simulink model "SimulationWithMotorAndGearbox"  (R2023a)
settings: configuration reference "SharedConfig" (kept outside this file)
undefined symbols (not defined in the file): Analyse, config_gearbox, config_motor, GB, gearbox_map, k_FW, motormap, motormap2
libraries: simulink x2
settings Model: PauseTimes=35  Creator=maximilian.tschochne  LastModifiedBy=ge49hus
settings ConfigSetRef: SourceName=SharedConfig  SourceLocation=Base Workspace

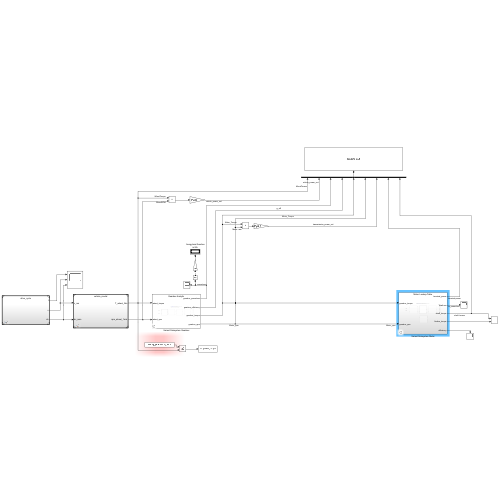
[thumbnail: Simulink's stored preview of the top-level diagram]
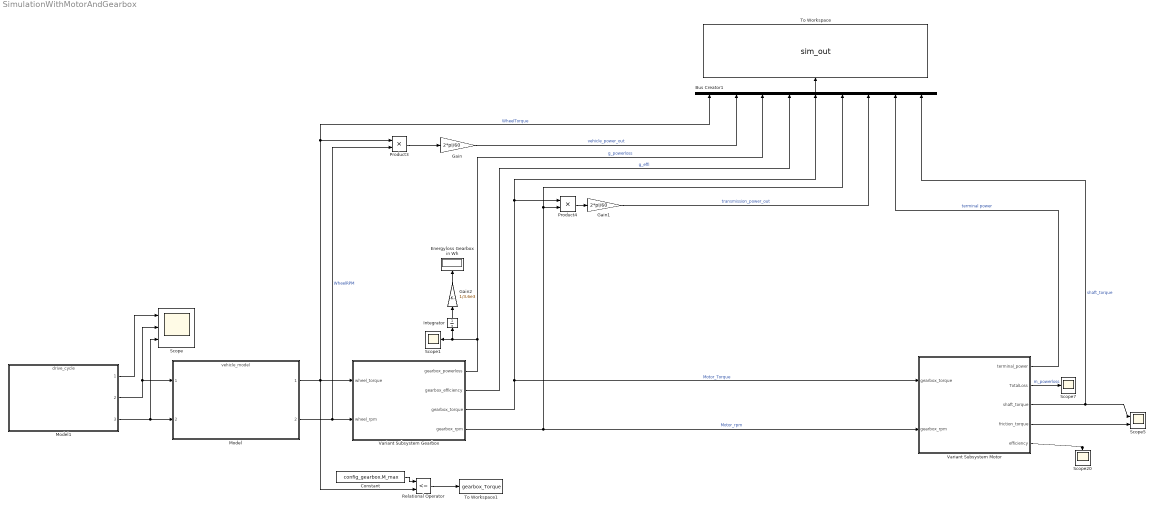
== system SimulationWithMotorAndGearbox ==
  Bus Creator1 : BusCreator  Inputs=9
  Constant : Constant  Value=config_gearbox.M_max
  Energyloss Gearbox in Wh : Display
  Gain : Gain  Gain=2*pi/60
  Gain1 : Gain  Gain=2*pi/60
  Gain2 : Gain  Gain=1/3.6e3
  Integrator : Integrator
  Model : ModelReference  ModelNameDialog=vehicle_model.slx  SimulationMode=Normal  ModelReferenceVersion=2.0
  Model1 : ModelReference  ModelNameDialog=drive_cycle.slx  SimulationMode=Normal  ModelReferenceVersion=1.0
  Product3 : Product
  Product4 : Product
  Relational Operator : RelationalOperator  Operator=<=  OutDataTypeStr=boolean  RndMeth=Simplest  InputSameDT=off
  Scope : Scope  NumInputPorts=3
  Scope1 : Scope
  Scope20 : Scope
  Scope5 : Scope  NumInputPorts=2
  Scope7 : Scope
  To Workspace : ToWorkspace  VariableName=sim_out  SaveFormat=Timeseries  SampleTime=-1
  To Workspace1 : ToWorkspace  VariableName=gearbox_Torque  SaveFormat=Timeseries  SampleTime=-1
  Variant Subsystem Gearbox : Subsystem  Variant=on
  Variant Subsystem Motor : Subsystem  Variant=on
  wires:
  Model1/1 -> Scope/1
  Model1/2 -> Scope/2, Model/1
  Model1/3 -> Scope/3, Model/2
  Bus Creator1/1 -> To Workspace/1
  Gain/1 -> Bus Creator1/2  "vehicle_power_out"
  Gain1/1 -> Bus Creator1/7  "transmission_power_out"
  Model/2 -> Product3/2, Variant Subsystem Gearbox/2(wheel_rpm)  "WheelRPM"
  Model/1 -> Variant Subsystem Gearbox/1(wheel_torque), Relational Operator/2, Bus Creator1/1, Product3/1  "WheelTorque"
  Product3/1 -> Gain/1
  Product4/1 -> Gain1/1
  Variant Subsystem Gearbox/1(gearbox_powerloss) -> Bus Creator1/3, Integrator/1, Scope1/1  "g_powerloss"
  Variant Subsystem Gearbox/2(gearbox_efficiency) -> Bus Creator1/4  "g_effi"
  Integrator/1 -> Gain2/1
  Gain2/1 -> Energyloss Gearbox in Wh/1
  Relational Operator/1 -> To Workspace1/1
  Constant/1 -> Relational Operator/1
  Variant Subsystem Gearbox/3(gearbox_torque) -> Bus Creator1/5, Product4/1, Variant Subsystem Motor/1(gearbox_torque)  "Motor_Torque"
  Variant Subsystem Gearbox/4(gearbox_rpm) -> Variant Subsystem Motor/2(gearbox_rpm), Bus Creator1/6, Product4/2  "Motor_rpm"
  Variant Subsystem Motor/3(shaft_torque) -> Bus Creator1/9, Scope5/1  "shaft_torque"
  Variant Subsystem Motor/5(efficiency) -> Scope20/1
  Variant Subsystem Motor/1(terminal_power) -> Bus Creator1/8  "terminal power"
  Variant Subsystem Motor/4(friction_torque) -> Scope5/2
  Variant Subsystem Motor/2(TotalLoss) -> Scope7/1  "m_powerloss"

== system SimulationWithMotorAndGearbox/Variant Subsystem Gearbox ==
  note: 1) Add Subsystem or Model blocks as valid variant choices.
      | 2) You cannot connect blocks at this level. At simulation, connectivity is automatically
      | determined, based on the active variant and port name matching.
  wheel_torque : Inport
  wheel_rpm : Inport  Port=2
  Gearbox Analytic : Subsystem  VariantControl="GB_Mode == \"Analytic\""
  Gearbox Const : Subsystem  VariantControl="GB_Mode == \"Const\""
  Gearbox Lookup-Table : Subsystem  VariantControl="GB_Mode == \"Lookup\""
  Gearbox Simple : Subsystem  VariantControl="GB_Mode == \"Simple\""
  gearbox_powerloss : Outport
  gearbox_efficiency : Outport  Port=2
  gearbox_torque : Outport  Port=3
  gearbox_rpm : Outport  Port=4

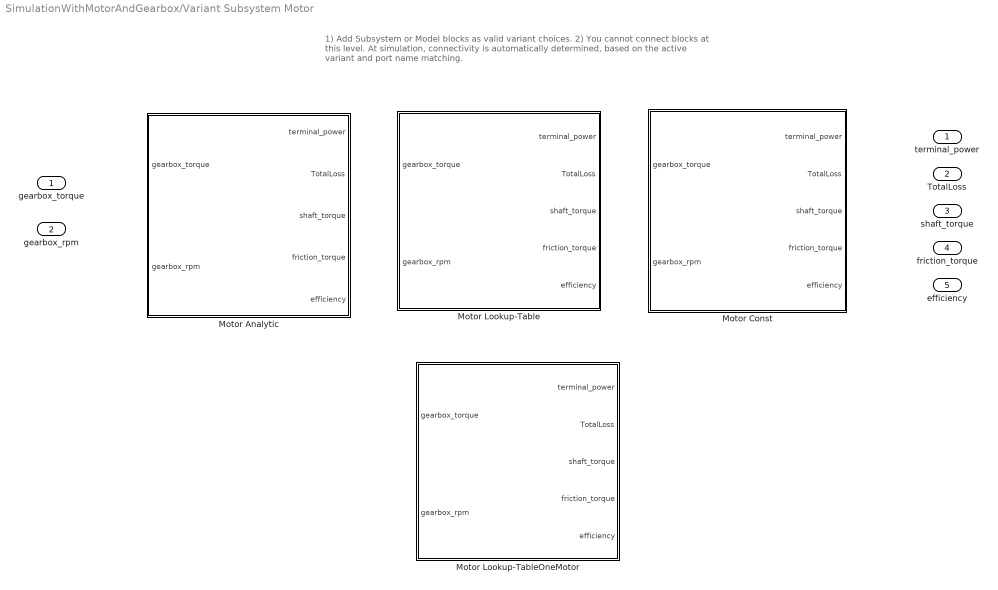
== system SimulationWithMotorAndGearbox/Variant Subsystem Motor ==
  note: 1) Add Subsystem or Model blocks as valid variant choices.
      | 2) You cannot connect blocks at this level. At simulation, connectivity is automatically
      | determined, based on the active variant and port name matching.
  gearbox_torque : Inport
  gearbox_rpm : Inport  Port=2
  Motor Analytic : Subsystem  VariantControl="Motor_Mode == \"Analytic\""
  Motor Const : Subsystem  VariantControl="Motor_Mode == \"Const\""
  Motor Lookup-Table : Subsystem  VariantControl="Motor_Mode == \"Lookup\""
  Motor Lookup-TableOneMotor : Subsystem  VariantControl="Motor_Mode == \"LookupOneMotor\""
  terminal_power : Outport
  TotalLoss : Outport  Port=2
  shaft_torque : Outport  Port=3
  friction_torque : Outport  Port=4
  efficiency : Outport  Port=5

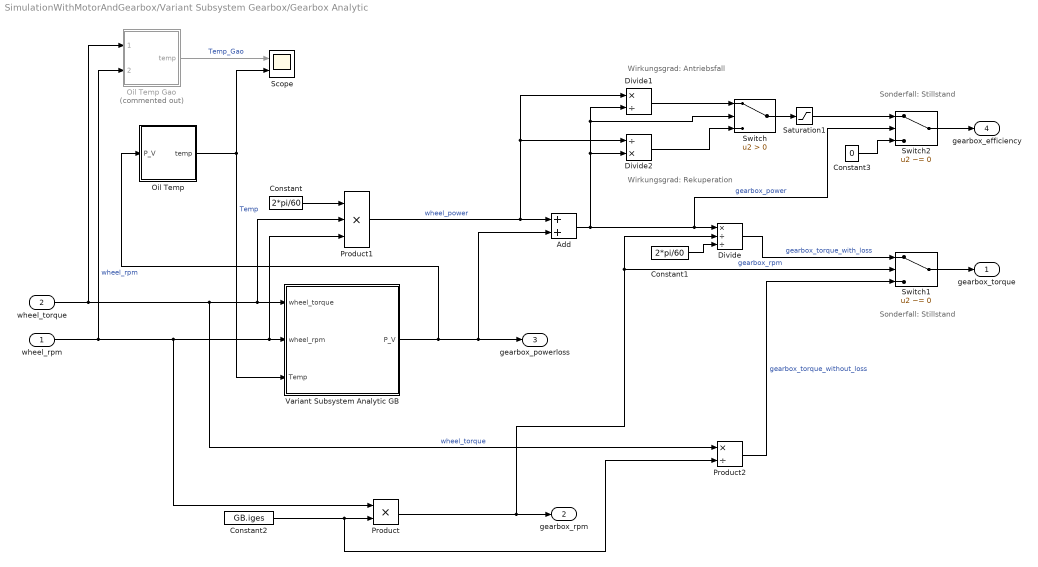
== system SimulationWithMotorAndGearbox/Variant Subsystem Gearbox/Gearbox Analytic ==
  note: Wirkungsgrad:
      | Antriebsfall
  note: Sonderfall: Stillstand
  note: Sonderfall: Stillstand
  note: Wirkungsgrad:
      | Rekuperation
  wheel_rpm : Inport
  wheel_torque : Inport  Port=2
  Add : Sum
  Constant : Constant  Value=2*pi/60
  Constant1 : Constant  Value=2*pi/60
  Constant2 : Constant  Value=GB.iges
  Constant3 : Constant  Value=0
  Divide : Product  Inputs=*//
  Divide1 : Product  Inputs=*/
  Divide2 : Product  Inputs=/*
  Oil Temp : Subsystem
  Oil Temp Gao : Subsystem  Commented=on
  Product : Product
  Product1 : Product  Inputs=3
  Product2 : Product  Inputs=*/
  Saturation1 : Saturate  UpperLimit=inf  LowerLimit=0
  Scope : Scope  NumInputPorts=2
  Switch : Switch  Criteria=u2 > Threshold  SaturateOnIntegerOverflow=off  InputSameDT=off
  Switch1 : Switch  Criteria=u2 ~= 0  SaturateOnIntegerOverflow=off  InputSameDT=off
  Switch2 : Switch  Criteria=u2 ~= 0  SaturateOnIntegerOverflow=off  InputSameDT=off
  Variant Subsystem Analytic GB : Subsystem  Variant=on
  gearbox_torque : Outport
  gearbox_rpm : Outport  Port=2
  gearbox_powerloss : Outport  Port=3
  gearbox_efficiency : Outport  Port=4
  wires:
  wheel_torque/1 -> Variant Subsystem Analytic GB/1(wheel_torque), Product1/2, Product2/1, Oil Temp Gao/1(T_wheel)  "wheel_torque"
  wheel_rpm/1 -> Product/1, Variant Subsystem Analytic GB/2(wheel_rpm), Product1/3, Oil Temp Gao/2(rpm_wheel)  "wheel_rpm"
  Variant Subsystem Analytic GB/1(P_V) -> Oil Temp/1(P_V), Add/2, gearbox_powerloss/1
  Constant2/1 -> Product2/2, Product/2
  Product/1 -> Switch1/2, Divide/2, gearbox_rpm/1  "gearbox_rpm"
  Constant/1 -> Product1/1
  Product1/1 -> Divide2/1, Divide1/1, Add/1  "wheel_power"
  Add/1 -> Divide2/2, Switch/2, Divide1/2, Switch2/2, Divide/1  "gearbox_power"
  Constant1/1 -> Divide/3
  Divide/1 -> Switch1/1  "gearbox_torque_with_loss"
  Switch/1 -> Saturation1/1
  Divide2/1 -> Switch/3
  Switch1/1 -> gearbox_torque/1
  Product2/1 -> Switch1/3  "gearbox_torque_without_loss"
  Switch2/1 -> gearbox_efficiency/1
  Constant3/1 -> Switch2/3
  Divide1/1 -> Switch/1
  Oil Temp Gao/1(temp) -> Scope/1  "Temp_Gao"
  Oil Temp/1(temp) -> Scope/2, Variant Subsystem Analytic GB/3(Temp)  "Temp"
  Saturation1/1 -> Switch2/1

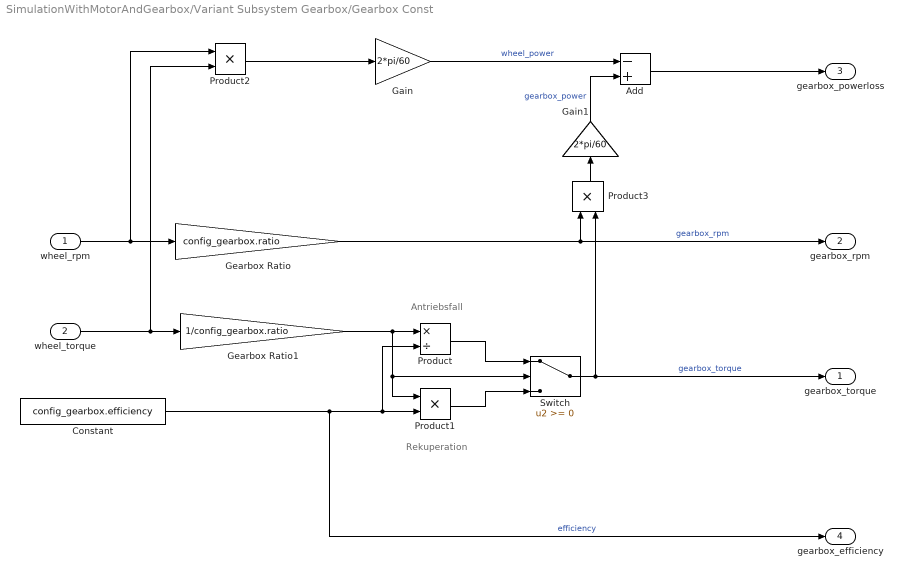
== system SimulationWithMotorAndGearbox/Variant Subsystem Gearbox/Gearbox Const ==
  note: Rekuperation
  note: Antriebsfall
  wheel_rpm : Inport
  wheel_torque : Inport  Port=2
  Add : Sum  Inputs=-+
  Constant : Constant  Value=config_gearbox.efficiency
  Gain : Gain  Gain=2*pi/60
  Gain1 : Gain  Gain=2*pi/60
  Gearbox Ratio : Gain  Gain=config_gearbox.ratio
  Gearbox Ratio1 : Gain  Gain=1/config_gearbox.ratio
  Product : Product  Inputs=*/
  Product1 : Product  Inputs=**
  Product2 : Product
  Product3 : Product
  Switch : Switch  SaturateOnIntegerOverflow=off  InputSameDT=off
  gearbox_torque : Outport
  gearbox_rpm : Outport  Port=2
  gearbox_powerloss : Outport  Port=3
  gearbox_efficiency : Outport  Port=4
  wires:
  wheel_rpm/1 -> Product2/1, Gearbox Ratio/1
  Gearbox Ratio/1 -> gearbox_rpm/1, Product3/1  "gearbox_rpm"
  wheel_torque/1 -> Product2/2, Gearbox Ratio1/1
  Gearbox Ratio1/1 -> Product1/1, Switch/2, Product/1
  Constant/1 -> gearbox_efficiency/1, Product1/2, Product/2  "efficiency"
  Product/1 -> Switch/1
  Product1/1 -> Switch/3
  Switch/1 -> gearbox_torque/1, Product3/2  "gearbox_torque"
  Product2/1 -> Gain/1
  Add/1 -> gearbox_powerloss/1
  Product3/1 -> Gain1/1
  Gain/1 -> Add/1  "wheel_power"
  Gain1/1 -> Add/2  "gearbox_power"

== system SimulationWithMotorAndGearbox/Variant Subsystem Gearbox/Gearbox Lookup-Table ==
  wheel_rpm : Inport
  wheel_torque : Inport  Port=2
  Oil Temp : Subsystem
  Oil Temp Gao : Subsystem  Commented=on
  Scope : Scope  Commented=on  NumInputPorts=2
  Variant Subsystem : Subsystem  Variant=on
  gearbox_torque : Outport
  gearbox_rpm : Outport  Port=2
  gearbox_powerloss : Outport  Port=3
  gearbox_efficiency : Outport  Port=4
  wires:
  Oil Temp Gao/1(temp) -> Scope/2
  wheel_torque/1 -> Oil Temp Gao/1(T_wheel), Variant Subsystem/1(wheel_torque)  "wheel_torque"
  wheel_rpm/1 -> Oil Temp Gao/2(rpm_wheel), Variant Subsystem/2(wheel_rpm)  "wheel_rpm"
  Variant Subsystem/4(gearbox_torque) -> gearbox_torque/1
  Variant Subsystem/1(loss_lockup) -> Oil Temp/1(P_V), gearbox_powerloss/1
  Variant Subsystem/3(gearbox_rpm) -> gearbox_rpm/1
  Variant Subsystem/2(gearbox_efficiency) -> gearbox_efficiency/1
  Oil Temp/1(temp) -> Scope/1, Variant Subsystem/3(Temp)

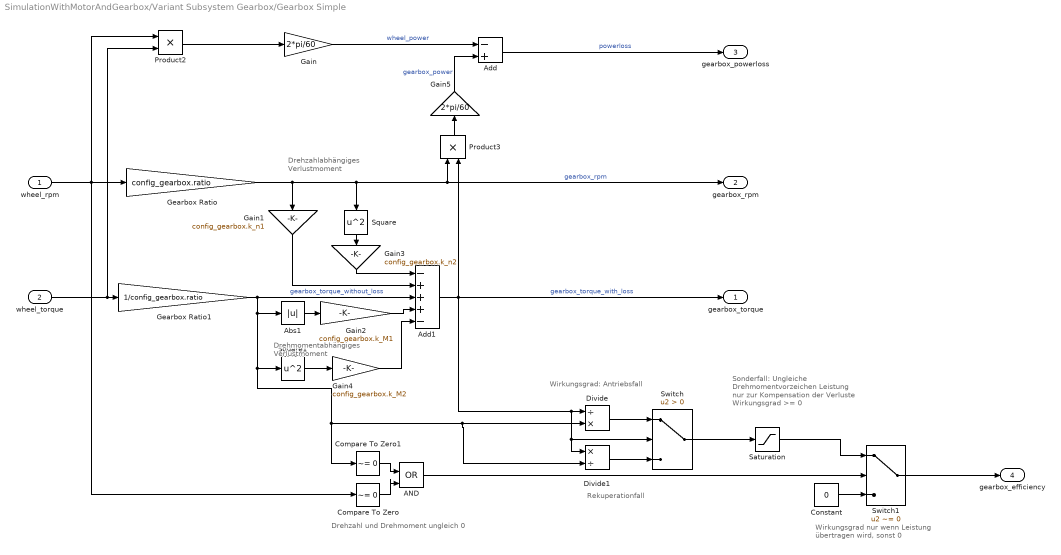
== system SimulationWithMotorAndGearbox/Variant Subsystem Gearbox/Gearbox Simple ==
  note: Rekuperationfall
  note: Sonderfall: Ungleiche Drehmomentvorzeichen
      | Leistung nur zur Kompensation der Verluste
      | Wirkungsgrad >= 0
  note: Drehzahl und Drehmoment ungleich 0
  note: Drehmomentabhängiges
      | Verlustmoment
  note: Drehzahlabhängiges
      | Verlustmoment
  note: Wirkungsgrad nur wenn Leistung
      | übertragen wird, sonst 0
  note: Wirkungsgrad: Antriebsfall
  wheel_rpm : Inport
  wheel_torque : Inport  Port=2
  AND : Logic  Operator=OR  IconShape=distinctive  AllPortsSameDT=off  OutDataTypeStr=boolean
  Abs1 : Abs  SaturateOnIntegerOverflow=off
  Add : Sum  Inputs=-+
  Add1 : Sum  Inputs=-+++-
  Compare To Zero : simulink/Logic and Bit Operations/Compare To Zero  relop=~=  OutDataTypeStr=boolean
  Compare To Zero1 : simulink/Logic and Bit Operations/Compare To Zero  relop=~=  OutDataTypeStr=boolean
  Constant : Constant  Value=0
  Divide : Product  Inputs=/*
  Divide1 : Product  Inputs=*/
  Gain : Gain  Gain=2*pi/60
  Gain1 : Gain  Gain=config_gearbox.k_n1
  Gain2 : Gain  Gain=config_gearbox.k_M1
  Gain3 : Gain  Gain=config_gearbox.k_n2
  Gain4 : Gain  Gain=config_gearbox.k_M2
  Gain5 : Gain  Gain=2*pi/60
  Gearbox Ratio : Gain  Gain=config_gearbox.ratio
  Gearbox Ratio1 : Gain  Gain=1/config_gearbox.ratio
  Product2 : Product
  Product3 : Product
  Saturation : Saturate  UpperLimit=inf  LowerLimit=0
  Square : Math  Operator=square
  Square1 : Math  Operator=square
  Switch : Switch  Criteria=u2 > Threshold  SaturateOnIntegerOverflow=off  InputSameDT=off
  Switch1 : Switch  Criteria=u2 ~= 0  SaturateOnIntegerOverflow=off  InputSameDT=off
  gearbox_torque : Outport
  gearbox_rpm : Outport  Port=2
  gearbox_powerloss : Outport  Port=3
  gearbox_efficiency : Outport  Port=4
  wires:
  Product3/1 -> Gain5/1
  Add/1 -> gearbox_powerloss/1  "powerloss"
  Add1/1 -> Product3/2, gearbox_torque/1, Switch/2, Divide1/1, Divide/1  "gearbox_torque_with_loss"
  wheel_torque/1 -> Product2/2, Gearbox Ratio1/1
  Gearbox Ratio/1 -> Square/1, Product3/1, gearbox_rpm/1, Gain1/1  "gearbox_rpm"
  wheel_rpm/1 -> Compare To Zero/1, Gearbox Ratio/1, Product2/1
  Gearbox Ratio1/1 -> Abs1/1, Square1/1, Compare To Zero1/1, Divide1/2, Divide/2, Add1/3  "gearbox_torque_without_loss"
  Gain1/1 -> Add1/2
  Gain2/1 -> Add1/4
  Abs1/1 -> Gain2/1
  Divide/1 -> Switch/1
  Switch/1 -> Saturation/1
  Divide1/1 -> Switch/3
  Constant/1 -> Switch1/3
  Gain3/1 -> Add1/1
  Square/1 -> Gain3/1
  Switch1/1 -> gearbox_efficiency/1
  Square1/1 -> Gain4/1
  Gain4/1 -> Add1/5
  Compare To Zero1/1 -> AND/1
  Compare To Zero/1 -> AND/2
  AND/1 -> Switch1/2
  Product2/1 -> Gain/1
  Gain/1 -> Add/1  "wheel_power"
  Gain5/1 -> Add/2  "gearbox_power"
  Saturation/1 -> Switch1/1

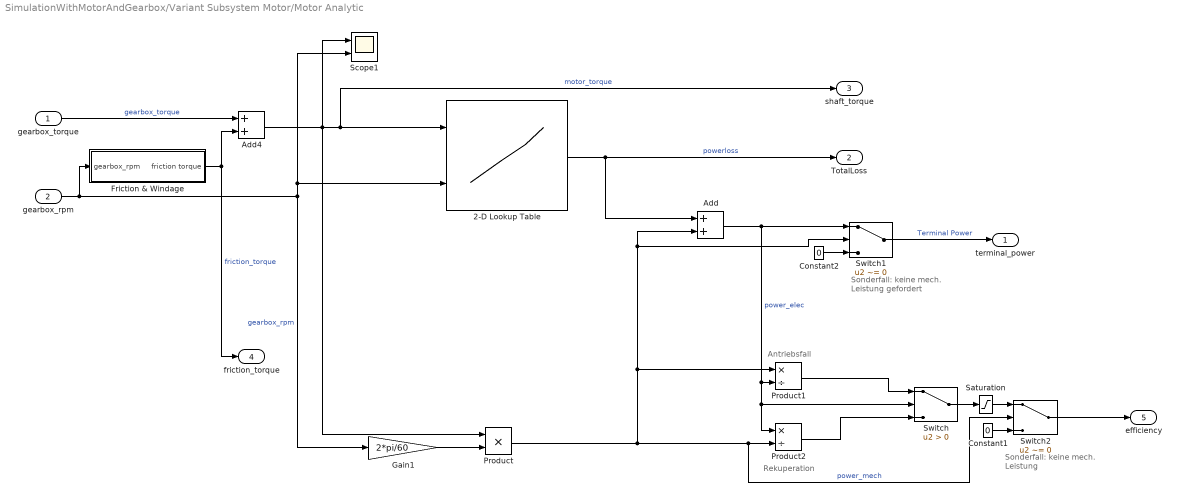
== system SimulationWithMotorAndGearbox/Variant Subsystem Motor/Motor Analytic ==
  note: Sonderfall:
      | keine mech. Leistung
  note: Antriebsfall
  note: Rekuperation
  note: Sonderfall: keine mech.
      | Leistung gefordert
  gearbox_torque : Inport
  gearbox_rpm : Inport  Port=2
  2-D Lookup Table : Lookup_n-D  BreakpointsForDimension1=Analyse.Betriebsdaten.M_vec(end:-1:1)  BreakpointsForDimension2=Analyse.Betriebsdaten.n_m_mesh(Analyse.Optionen.M_tics,:)  Table=Analyse.Verluste.P_vges_mesh(end:-1:1,:)  InternalRulePriority=Speed  RndMeth=Simplest
      settings: InputPortMap=u0,u1
  Add : Sum
  Add4 : Sum
  Constant1 : Constant  Value=0
  Constant2 : Constant  Value=0
  Friction & Windage : Subsystem
  Gain1 : Gain  Gain=2*pi/60
  Product : Product
  Product1 : Product  Inputs=*/
  Product2 : Product  Inputs=*/
  Saturation : Saturate  UpperLimit=inf  LowerLimit=0
  Scope1 : Scope  NumInputPorts=2
  Switch : Switch  Criteria=u2 > Threshold  SaturateOnIntegerOverflow=off  InputSameDT=off
  Switch1 : Switch  Criteria=u2 ~= 0  SaturateOnIntegerOverflow=off  InputSameDT=off
  Switch2 : Switch  Criteria=u2 ~= 0  SaturateOnIntegerOverflow=off  InputSameDT=off
  terminal_power : Outport
  TotalLoss : Outport  Port=2
  shaft_torque : Outport  Port=3
  friction_torque : Outport  Port=4
  efficiency : Outport  Port=5
  wires:
  gearbox_rpm/1 -> Friction & Windage/1(gearbox_rpm), Scope1/2, 2-D Lookup Table/2, Gain1/1  "gearbox_rpm"
  2-D Lookup Table/1 -> Add/1, TotalLoss/1  "powerloss"
  Product/1 -> Switch2/2, Product2/2, Switch1/2, Add/2, Product1/1  "power_mech"
  Add/1 -> Switch1/1, Product2/1, Switch/2, Product1/2  "power_elec"
  Product2/1 -> Switch/3
  Add4/1 -> Scope1/1, Product/1, shaft_torque/1, 2-D Lookup Table/1  "motor_torque"
  Switch2/1 -> efficiency/1
  Gain1/1 -> Product/2
  Constant2/1 -> Switch1/3
  Switch1/1 -> terminal_power/1  "Terminal Power"
  Product1/1 -> Switch/1
  gearbox_torque/1 -> Add4/1  "gearbox_torque"
  Friction & Windage/1(friction torque) -> friction_torque/1, Add4/2  "friction_torque"
  Switch/1 -> Saturation/1
  Constant1/1 -> Switch2/3
  Saturation/1 -> Switch2/1

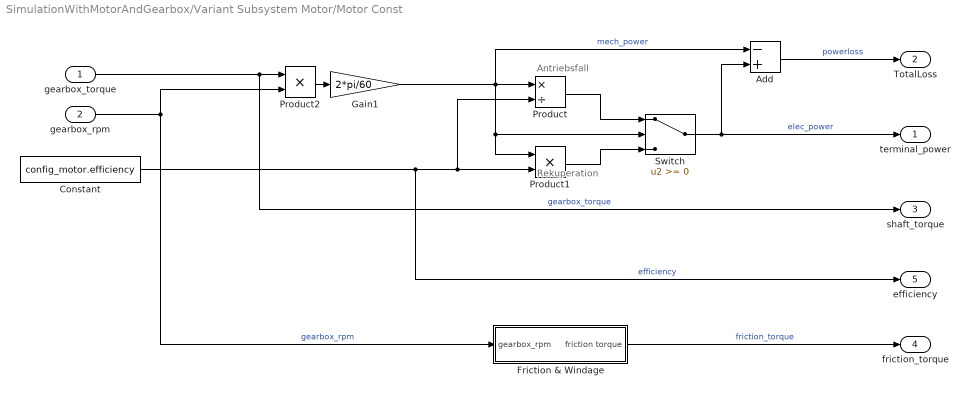
== system SimulationWithMotorAndGearbox/Variant Subsystem Motor/Motor Const ==
  note: Rekuperation
  note: Antriebsfall
  gearbox_torque : Inport
  gearbox_rpm : Inport  Port=2
  Add : Sum  Inputs=-+
  Constant : Constant  Value=config_motor.efficiency
  Friction & Windage : Subsystem
  Gain1 : Gain  Gain=2*pi/60
  Product : Product  Inputs=*/
  Product1 : Product  Inputs=**
  Product2 : Product
  Switch : Switch  SaturateOnIntegerOverflow=off  InputSameDT=off
  terminal_power : Outport
  TotalLoss : Outport  Port=2
  shaft_torque : Outport  Port=3
  friction_torque : Outport  Port=4
  efficiency : Outport  Port=5
  wires:
  Product2/1 -> Gain1/1
  Constant/1 -> efficiency/1, Product1/2, Product/2  "efficiency"
  Product/1 -> Switch/1
  Product1/1 -> Switch/3
  Add/1 -> TotalLoss/1  "powerloss"
  Switch/1 -> terminal_power/1, Add/2  "elec_power"
  gearbox_rpm/1 -> Friction & Windage/1(gearbox_rpm), Product2/2  "gearbox_rpm"
  Gain1/1 -> Add/1, Product1/1, Switch/2, Product/1  "mech_power"
  gearbox_torque/1 -> Product2/1, shaft_torque/1  "gearbox_torque"
  Friction & Windage/1(friction torque) -> friction_torque/1  "friction_torque"

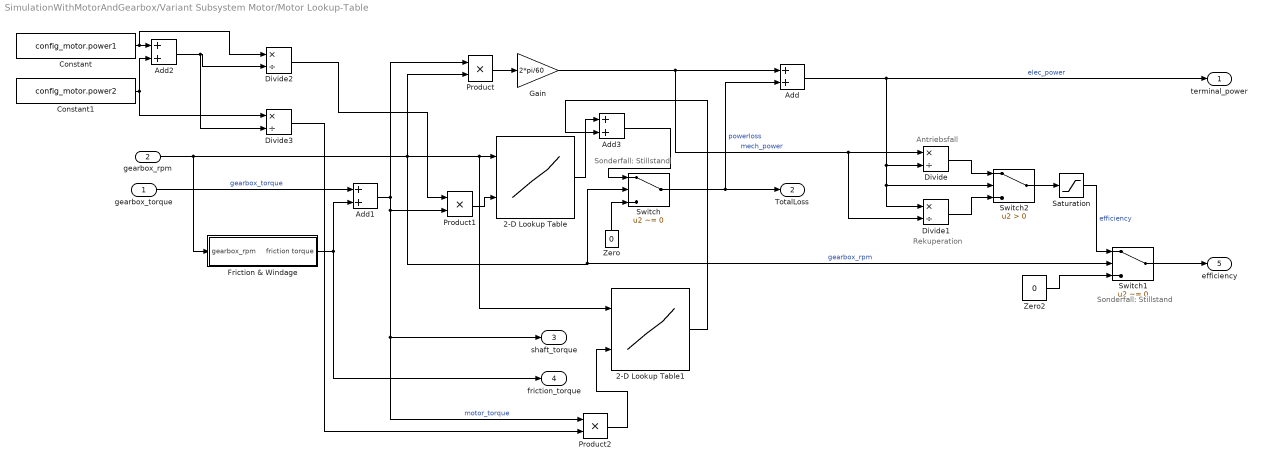
== system SimulationWithMotorAndGearbox/Variant Subsystem Motor/Motor Lookup-Table ==
  note: Sonderfall: Stillstand
  note: Rekuperation
  note: Antriebsfall
  note: Sonderfall: Stillstand
  gearbox_torque : Inport
  gearbox_rpm : Inport  Port=2
  2-D Lookup Table : Lookup_n-D  BreakpointsForDimension1=motormap.nVec  BreakpointsForDimension2=motormap.MVec  Table=motormap.Loss  InternalRulePriority=Speed  RndMeth=Simplest
      settings: InputPortMap=u0,u1
  2-D Lookup Table1 : Lookup_n-D  BreakpointsForDimension1=motormap2.nVec  BreakpointsForDimension2=motormap2.MVec  Table=motormap2.Loss  InternalRulePriority=Speed  RndMeth=Simplest
      settings: InputPortMap=u0,u1
  Add{,1..3} (4 alike) : Sum
  Constant : Constant  Value=config_motor.power1
  Constant1 : Constant  Value=config_motor.power2
  Divide{,1..3} (4 alike) : Product  Inputs=*/
  Friction & Windage : Subsystem
  Gain : Gain  Gain=2*pi/60
  Product : Product
  Product1 : Product
  Product2 : Product
  Saturation : Saturate  UpperLimit=inf  LowerLimit=0
  Switch : Switch  Criteria=u2 ~= 0  Threshold=1  SaturateOnIntegerOverflow=off  InputSameDT=off
  Switch1 : Switch  Criteria=u2 ~= 0  SaturateOnIntegerOverflow=off  InputSameDT=off
  Switch2 : Switch  Criteria=u2 > Threshold  SaturateOnIntegerOverflow=off  InputSameDT=off
  Zero : Constant  Value=0  OutDataTypeStr=Inherit: Inherit via back propagation
  Zero2 : Constant  Value=0  OutDataTypeStr=Inherit: Inherit via back propagation
  terminal_power : Outport
  TotalLoss : Outport  Port=2
  shaft_torque : Outport  Port=3
  friction_torque : Outport  Port=4
  efficiency : Outport  Port=5
  wires:
  gearbox_torque/1 -> Add1/1  "gearbox_torque"
  2-D Lookup Table/1 -> Add3/1
  Product/1 -> Gain/1
  Gain/1 -> Divide/1, Divide1/2, Add/1  "mech_power"
  Switch/1 -> TotalLoss/1, Add/2  "powerloss"
  Zero/1 -> Switch/3
  Add/1 -> Switch2/2, Divide1/1, Divide/2, terminal_power/1  "elec_power"
  Switch1/1 -> efficiency/1
  Zero2/1 -> Switch1/3
  Switch2/1 -> Saturation/1
  Divide/1 -> Switch2/1
  Divide1/1 -> Switch2/3
  Saturation/1 -> Switch1/1  "efficiency"
  gearbox_rpm/1 -> 2-D Lookup Table1/1, 2-D Lookup Table/1, Switch1/2, Switch/2, Product/2, Friction & Windage/1(gearbox_rpm)  "gearbox_rpm"
  Add1/1 -> Product1/2, Product2/1, shaft_torque/1, Product/1  "motor_torque"
  Friction & Windage/1(friction torque) -> Add1/2, friction_torque/1
  Constant/1 -> Divide2/1, Add2/1
  Constant1/1 -> Add2/2, Divide3/1
  Add2/1 -> Divide3/2, Divide2/2
  Divide2/1 -> Product1/1
  Product1/1 -> 2-D Lookup Table/2
  Product2/1 -> 2-D Lookup Table1/2
  Divide3/1 -> Product2/2
  2-D Lookup Table1/1 -> Add3/2
  Add3/1 -> Switch/1

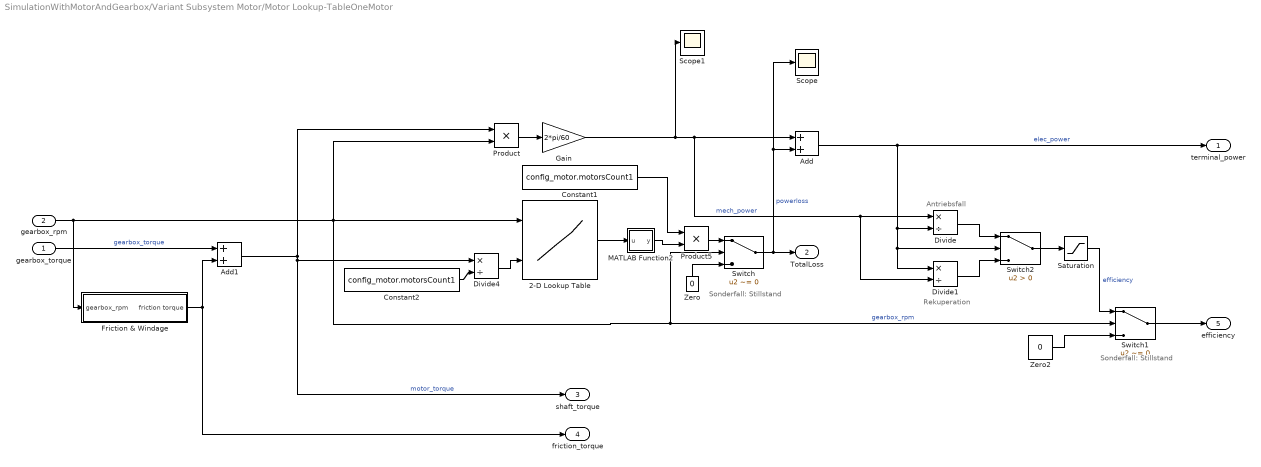
== system SimulationWithMotorAndGearbox/Variant Subsystem Motor/Motor Lookup-TableOneMotor ==
  note: Sonderfall: Stillstand
  note: Rekuperation
  note: Antriebsfall
  note: Sonderfall: Stillstand
  gearbox_torque : Inport
  gearbox_rpm : Inport  Port=2
  2-D Lookup Table : Lookup_n-D  BreakpointsForDimension1=motormap.nVec  BreakpointsForDimension2=motormap.MVec  Table=motormap.Loss  InternalRulePriority=Speed  RndMeth=Simplest
      settings: InputPortMap=u0,u1
  Add : Sum
  Add1 : Sum
  Constant1 : Constant  Value=config_motor.motorsCount1
  Constant2 : Constant  Value=config_motor.motorsCount1
  Divide : Product  Inputs=*/
  Divide1 : Product  Inputs=*/
  Divide4 : Product  Inputs=*/
  Friction & Windage : Subsystem
  Gain : Gain  Gain=2*pi/60
  MATLAB Function2 : MATLAB Function  TreatAsAtomicUnit=on
  Product : Product
  Product5 : Product
  Saturation : Saturate  UpperLimit=inf  LowerLimit=0
  Scope : Scope
  Scope1 : Scope
  Switch : Switch  Criteria=u2 ~= 0  Threshold=1  SaturateOnIntegerOverflow=off  InputSameDT=off
  Switch1 : Switch  Criteria=u2 ~= 0  SaturateOnIntegerOverflow=off  InputSameDT=off
  Switch2 : Switch  Criteria=u2 > Threshold  SaturateOnIntegerOverflow=off  InputSameDT=off
  Zero : Constant  Value=0  OutDataTypeStr=Inherit: Inherit via back propagation
  Zero2 : Constant  Value=0  OutDataTypeStr=Inherit: Inherit via back propagation
  terminal_power : Outport
  TotalLoss : Outport  Port=2
  shaft_torque : Outport  Port=3
  friction_torque : Outport  Port=4
  efficiency : Outport  Port=5
  wires:
  gearbox_torque/1 -> Add1/1  "gearbox_torque"
  Product/1 -> Gain/1
  Gain/1 -> Scope1/1, Divide/1, Divide1/2, Add/1  "mech_power"
  Switch/1 -> Add/2, Scope/1, TotalLoss/1  "powerloss"
  Zero/1 -> Switch/3
  Add/1 -> Switch2/2, Divide1/1, Divide/2, terminal_power/1  "elec_power"
  Switch1/1 -> efficiency/1
  Zero2/1 -> Switch1/3
  Switch2/1 -> Saturation/1
  Divide/1 -> Switch2/1
  Divide1/1 -> Switch2/3
  Saturation/1 -> Switch1/1  "efficiency"
  gearbox_rpm/1 -> 2-D Lookup Table/1, Switch1/2, Switch/2, Product/2, Friction & Windage/1(gearbox_rpm)  "gearbox_rpm"
  Add1/1 -> Divide4/1, shaft_torque/1, Product/1  "motor_torque"
  Friction & Windage/1(friction torque) -> friction_torque/1, Add1/2
  2-D Lookup Table/1 -> MATLAB Function2/1(u)
  MATLAB Function2/1(y) -> Product5/2
  Divide4/1 -> 2-D Lookup Table/2
  Product5/1 -> Switch/1
  Constant2/1 -> Divide4/2
  Constant1/1 -> Product5/1

== system SimulationWithMotorAndGearbox/Variant Subsystem Gearbox/Gearbox Analytic/Oil Temp ==
  P_V : Inport
  IC : InitialCondition  Value=25
  MATLAB Function : MATLAB Function  TreatAsAtomicUnit=on
  Memory1 : Memory  InitialCondition=config_vehicle.ambient_temp - 273
  Memory2 : Memory  InitialCondition=config_vehicle.ambient_temp - 273
  Scope : Scope
  temp : Outport
  wires:
  MATLAB Function/1(T) -> IC/1  "GB_temp"
  Memory1/1 -> MATLAB Function/1(t)
  P_V/1 -> Memory2/1
  IC/1 -> Scope/1, Memory1/1, temp/1
  Memory2/1 -> MATLAB Function/2(P_V)

== system SimulationWithMotorAndGearbox/Variant Subsystem Gearbox/Gearbox Analytic/Oil Temp Gao ==
  note: entspricht 2pi/60 * 1e-3
  T_wheel : Inport
  rpm_wheel : Inport  Port=2
  MATLAB Function : MATLAB Function  TreatAsAtomicUnit=on
  Memory1 : Memory  InitialCondition=config_vehicle.ambient_temp - 273
  Multiply5 : Gain  Gain=1/9550
  Product2 : Product
  Scope : Scope
  temp : Outport
  wires:
  Product2/1 -> Multiply5/1
  rpm_wheel/1 -> MATLAB Function/3(rpm), Product2/2
  T_wheel/1 -> Product2/1
  MATLAB Function/1(T) -> Scope/1, Memory1/1, temp/1
  Memory1/1 -> MATLAB Function/1(t)
  Multiply5/1 -> MATLAB Function/2(P)

== system SimulationWithMotorAndGearbox/Variant Subsystem Gearbox/Gearbox Analytic/Variant Subsystem Analytic GB ==
  note: 1) Add Subsystem or Model blocks as valid variant choices.
      | 2) You cannot connect blocks at this level. At simulation, connectivity is automatically
      | determined, based on the active variant and port name matching.
  wheel_torque : Inport
  wheel_rpm : Inport  Port=2
  Temp : Inport  Port=3
  Einstufig_Achsparallel : Subsystem  VariantControl=GB_Stufen == 1
  Zweistufig_Achsparallel : Subsystem  VariantControl="GB_Stufen == 2 && GB_Topology == \"achsparallel\""
  Zweistufig_Koaxial : Subsystem  VariantControl="GB_Stufen == 2 && GB_Topology == \"koaxial\""
  P_V : Outport

== system SimulationWithMotorAndGearbox/Variant Subsystem Gearbox/Gearbox Lookup-Table/Oil Temp ==
  P_V : Inport
  IC : InitialCondition  Value=25
  MATLAB Function : MATLAB Function  TreatAsAtomicUnit=on
  Memory1 : Memory  InitialCondition=config_vehicle.ambient_temp - 273
  Memory2 : Memory  InitialCondition=config_vehicle.ambient_temp - 273
  Scope : Scope
  temp : Outport
  wires:
  MATLAB Function/1(T) -> IC/1  "GB_temp"
  Memory1/1 -> MATLAB Function/1(t)
  P_V/1 -> Memory2/1
  IC/1 -> Scope/1, Memory1/1, temp/1
  Memory2/1 -> MATLAB Function/2(P_V)

== system SimulationWithMotorAndGearbox/Variant Subsystem Gearbox/Gearbox Lookup-Table/Oil Temp Gao ==
  note: entspricht 2pi/60 * 1e-3
  T_wheel : Inport
  rpm_wheel : Inport  Port=2
  MATLAB Function : MATLAB Function  TreatAsAtomicUnit=on
  Memory1 : Memory  InitialCondition=config_vehicle.ambient_temp - 273
  Multiply5 : Gain  Gain=1/9550
  Product2 : Product
  Scope : Scope
  temp : Outport
  wires:
  Product2/1 -> Multiply5/1
  rpm_wheel/1 -> MATLAB Function/3(rpm), Product2/2
  T_wheel/1 -> Product2/1
  MATLAB Function/1(T) -> Scope/1, Memory1/1, temp/1
  Memory1/1 -> MATLAB Function/1(t)
  Multiply5/1 -> MATLAB Function/2(P)

== system SimulationWithMotorAndGearbox/Variant Subsystem Gearbox/Gearbox Lookup-Table/Variant Subsystem ==
  note: 1) Add Subsystem or Model blocks as valid variant choices.
      | 2) You cannot connect blocks at this level. At simulation, connectivity is automatically
      | determined, based on the active variant and port name matching.
  wheel_torque : Inport
  wheel_rpm : Inport  Port=2
  Temp : Inport  Port=3
  ETA_map : Subsystem  VariantControl="gearbox_map.map_type == \"Eta\""
  LOSS_map : Subsystem  VariantControl="gearbox_map.map_type == \"Loss\""
  loss_lockup : Outport
  gearbox_efficiency : Outport  Port=2
  gearbox_rpm : Outport  Port=3
  gearbox_torque : Outport  Port=4

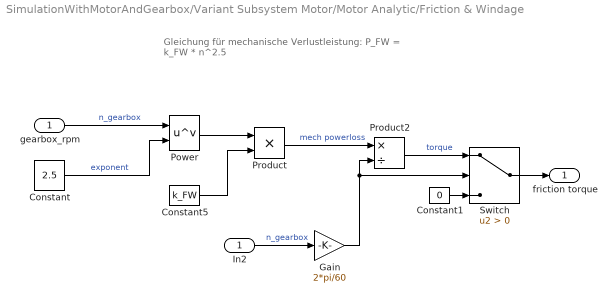
== system SimulationWithMotorAndGearbox/Variant Subsystem Motor/Motor Analytic/Friction & Windage ==
  note: Gleichung für mechanische Verlustleistung:
      | P_FW = k_FW * n^2.5
  gearbox_rpm : Inport
  Constant : Constant  Value=2.5
  Constant1 : Constant  Value=0
  Constant5 : Constant  Value=k_FW
  Gain : Gain  Gain=2*pi/60
  In2 : InportShadow
  Power : Math  Operator=pow
  Product : Product
  Product2 : Product  Inputs=*/
  Switch : Switch  Criteria=u2 > Threshold  SaturateOnIntegerOverflow=off  InputSameDT=off
  friction torque : Outport
  wires:
  gearbox_rpm/1 -> Power/1  "n_gearbox"
  Constant/1 -> Power/2  "exponent"
  Power/1 -> Product/1
  Constant5/1 -> Product/2
  Product/1 -> Product2/1  "mech powerloss"
  Product2/1 -> Switch/1  "torque"
  In2/1 -> Gain/1  "n_gearbox"
  Gain/1 -> Product2/2, Switch/2
  Switch/1 -> friction torque/1
  Constant1/1 -> Switch/3

== system SimulationWithMotorAndGearbox/Variant Subsystem Motor/Motor Const/Friction & Windage ==
  note: Gleichung für mechanische Verlustleistung:
      | P_FW = k_FW * n^2.5
  gearbox_rpm : Inport
  Constant : Constant  Value=2.5
  Constant1 : Constant  Value=0
  Constant5 : Constant  Value=k_FW
  Gain : Gain  Gain=2*pi/60
  In2 : InportShadow
  Power : Math  Operator=pow
  Product : Product
  Product2 : Product  Inputs=*/
  Switch : Switch  Criteria=u2 > Threshold  SaturateOnIntegerOverflow=off  InputSameDT=off
  friction torque : Outport
  wires:
  gearbox_rpm/1 -> Power/1  "n_gearbox"
  Constant/1 -> Power/2  "exponent"
  Power/1 -> Product/1
  Constant5/1 -> Product/2
  Product/1 -> Product2/1  "mech powerloss"
  Product2/1 -> Switch/1  "torque"
  In2/1 -> Gain/1  "n_gearbox"
  Gain/1 -> Product2/2, Switch/2
  Switch/1 -> friction torque/1
  Constant1/1 -> Switch/3

== system SimulationWithMotorAndGearbox/Variant Subsystem Motor/Motor Lookup-Table/Friction & Windage ==
  note: Gleichung für mechanische Verlustleistung:
      | P_FW = k_FW * n^2.5
  gearbox_rpm : Inport
  Constant : Constant  Value=2.5
  Constant1 : Constant  Value=0
  Constant5 : Constant  Value=k_FW
  Gain : Gain  Gain=2*pi/60
  In2 : InportShadow
  Power : Math  Operator=pow
  Product : Product
  Product2 : Product  Inputs=*/
  Switch : Switch  Criteria=u2 > Threshold  SaturateOnIntegerOverflow=off  InputSameDT=off
  friction torque : Outport
  wires:
  gearbox_rpm/1 -> Power/1  "n_gearbox"
  Constant/1 -> Power/2  "exponent"
  Power/1 -> Product/1
  Constant5/1 -> Product/2
  Product/1 -> Product2/1  "mech powerloss"
  Product2/1 -> Switch/1  "torque"
  In2/1 -> Gain/1  "n_gearbox"
  Gain/1 -> Product2/2, Switch/2
  Switch/1 -> friction torque/1
  Constant1/1 -> Switch/3

== system SimulationWithMotorAndGearbox/Variant Subsystem Motor/Motor Lookup-TableOneMotor/Friction & Windage ==
  note: Gleichung für mechanische Verlustleistung:
      | P_FW = k_FW * n^2.5
  gearbox_rpm : Inport
  Constant : Constant  Value=2.5
  Constant1 : Constant  Value=0
  Constant5 : Constant  Value=k_FW
  Gain : Gain  Gain=2*pi/60
  In2 : InportShadow
  Power : Math  Operator=pow
  Product : Product
  Product2 : Product  Inputs=*/
  Switch : Switch  Criteria=u2 > Threshold  SaturateOnIntegerOverflow=off  InputSameDT=off
  friction torque : Outport
  wires:
  gearbox_rpm/1 -> Power/1  "n_gearbox"
  Constant/1 -> Power/2  "exponent"
  Power/1 -> Product/1
  Constant5/1 -> Product/2
  Product/1 -> Product2/1  "mech powerloss"
  Product2/1 -> Switch/1  "torque"
  In2/1 -> Gain/1  "n_gearbox"
  Gain/1 -> Product2/2, Switch/2
  Switch/1 -> friction torque/1
  Constant1/1 -> Switch/3

== system SimulationWithMotorAndGearbox/Variant Subsystem Gearbox/Gearbox Analytic/Variant Subsystem Analytic GB/Einstufig_Achsparallel ==
  wheel_torque : Inport
  wheel_rpm : Inport  Port=2
  Temp : Inport  Port=3
  Add : Sum
  MATLAB Function : MATLAB Function  TreatAsAtomicUnit=on
  Ölpumpe : Subsystem
  P_V : Outport
  wires:
  wheel_rpm/1 -> Ölpumpe/1(nrad), MATLAB Function/2(nrad)
  MATLAB Function/1(P_V) -> Add/1
  wheel_torque/1 -> MATLAB Function/1(Mrad)
  Temp/1 -> MATLAB Function/3(Temp)
  Add/1 -> P_V/1
  Ölpumpe/1(power_oilpump) -> Add/2

== system SimulationWithMotorAndGearbox/Variant Subsystem Gearbox/Gearbox Analytic/Variant Subsystem Analytic GB/Zweistufig_Achsparallel ==
  wheel_torque : Inport
  wheel_rpm : Inport  Port=2
  Temp : Inport  Port=3
  Add : Sum
  MATLAB Function : MATLAB Function  TreatAsAtomicUnit=on
  Ölpumpe : Subsystem
  P_V : Outport
  wires:
  wheel_rpm/1 -> Ölpumpe/1(nrad), MATLAB Function/2(nrad)
  MATLAB Function/1(P_V) -> Add/1
  wheel_torque/1 -> MATLAB Function/1(Mrad)
  Temp/1 -> MATLAB Function/3(Temp)
  Add/1 -> P_V/1
  Ölpumpe/1(power_oilpump) -> Add/2

== system SimulationWithMotorAndGearbox/Variant Subsystem Gearbox/Gearbox Analytic/Variant Subsystem Analytic GB/Zweistufig_Koaxial ==
  wheel_torque : Inport
  wheel_rpm : Inport  Port=2
  Temp : Inport  Port=3
  Add : Sum
  MATLAB Function : MATLAB Function  TreatAsAtomicUnit=on
  Ölpumpe : Subsystem
  P_V : Outport
  wires:
  Temp/1 -> MATLAB Function/3(Temp)
  wheel_torque/1 -> MATLAB Function/1(Mrad)
  MATLAB Function/1(P_V) -> Add/1
  wheel_rpm/1 -> Ölpumpe/1(nrad), MATLAB Function/2(nrad)
  Add/1 -> P_V/1
  Ölpumpe/1(power_oilpump) -> Add/2

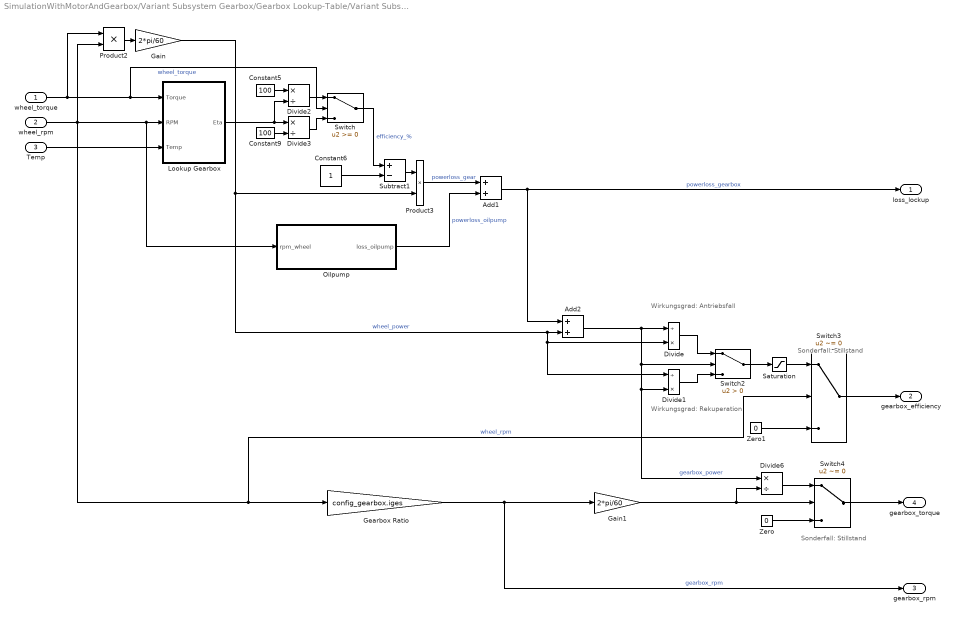
== system SimulationWithMotorAndGearbox/Variant Subsystem Gearbox/Gearbox Lookup-Table/Variant Subsystem/ETA_map ==
  note: Sonderfall: Stillstand
  note: Sonderfall: Stillstand
  note: Wirkungsgrad:
      | Antriebsfall
  note: Wirkungsgrad:
      | Rekuperation
  wheel_torque : Inport
  wheel_rpm : Inport  Port=2
  Temp : Inport  Port=3
  Add1 : Sum
  Add2 : Sum
  Constant5 : Constant  Value=100
  Constant6 : Constant
  Constant9 : Constant  Value=100
  Divide : Product  Inputs=/*
  Divide1 : Product  Inputs=/*
  Divide2 : Product  Inputs=*/
  Divide3 : Product  Inputs=*/
  Divide6 : Product  Inputs=*/
  Gain : Gain  Gain=2*pi/60
  Gain1 : Gain  Gain=2*pi/60
  Gearbox Ratio : Gain  Gain=config_gearbox.iges
  Lookup Gearbox : Subsystem  Variant=on
  Oilpump : Subsystem
  Product2 : Product  Inputs=**
  Product3 : Product  Inputs=**
  Saturation : Saturate  UpperLimit=inf  LowerLimit=0
  Subtract1 : Sum  Inputs=+-
  Switch : Switch  SaturateOnIntegerOverflow=off  InputSameDT=off
  Switch2 : Switch  Criteria=u2 > Threshold  SaturateOnIntegerOverflow=off  InputSameDT=off
  Switch3 : Switch  Criteria=u2 ~= 0  SaturateOnIntegerOverflow=off  InputSameDT=off
  Switch4 : Switch  Criteria=u2 ~= 0  SaturateOnIntegerOverflow=off  InputSameDT=off
  Zero : Constant  Value=0  OutDataTypeStr=Inherit: Inherit via back propagation
  Zero1 : Constant  Value=0  OutDataTypeStr=Inherit: Inherit via back propagation
  loss_lockup : Outport
  gearbox_efficiency : Outport  Port=2
  gearbox_rpm : Outport  Port=3
  gearbox_torque : Outport  Port=4
  wires:
  wheel_torque/1 -> Lookup Gearbox/1(Torque), Switch/2, Product2/1  "wheel_torque"
  Divide1/1 -> Switch2/3
  Product2/1 -> Gain/1
  wheel_rpm/1 -> Switch3/2, Gearbox Ratio/1, Product2/2, Oilpump/1(rpm_wheel), Lookup Gearbox/2(RPM)  "wheel_rpm"
  Constant6/1 -> Subtract1/2
  Subtract1/1 -> Product3/1
  Switch/1 -> Subtract1/1  "efficiency_%"
  Product3/1 -> Add1/1  "powerloss_gear"
  Zero1/1 -> Switch3/3
  Switch2/1 -> Saturation/1
  Divide2/1 -> Switch/1
  Zero/1 -> Switch4/3
  Switch4/1 -> gearbox_torque/1
  Switch3/1 -> gearbox_efficiency/1
  Divide6/1 -> Switch4/1
  Gearbox Ratio/1 -> Gain1/1, gearbox_rpm/1  "gearbox_rpm"
  Divide3/1 -> Switch/3
  Add2/1 -> Switch2/2, Divide6/1, Divide1/2, Divide/1  "gearbox_power"
  Gain1/1 -> Switch4/2, Divide6/2
  Temp/1 -> Lookup Gearbox/3(Temp)
  Gain/1 -> Product3/2, Divide1/1, Divide/2, Add2/2  "wheel_power"
  Add1/1 -> Add2/1, loss_lockup/1  "powerloss_gearbox"
  Constant9/1 -> Divide3/2
  Oilpump/1(loss_oilpump) -> Add1/2  "powerloss_oilpump"
  Lookup Gearbox/1(Eta) -> Divide2/2, Divide3/1
  Divide/1 -> Switch2/1
  Constant5/1 -> Divide2/1
  Saturation/1 -> Switch3/1

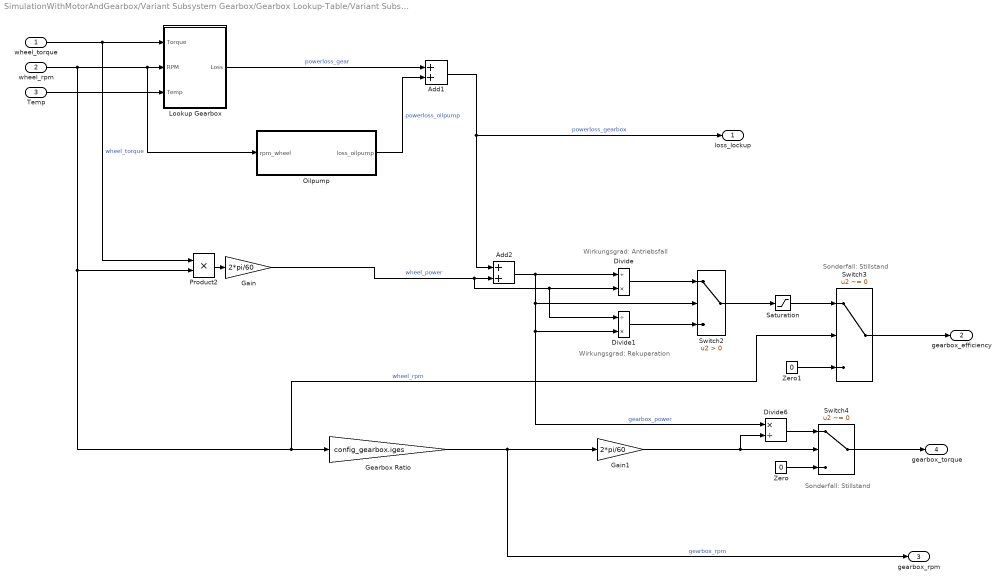
== system SimulationWithMotorAndGearbox/Variant Subsystem Gearbox/Gearbox Lookup-Table/Variant Subsystem/LOSS_map ==
  note: Sonderfall: Stillstand
  note: Wirkungsgrad: Antriebsfall
  note: Wirkungsgrad: Rekuperation
  note: Sonderfall: Stillstand
  wheel_torque : Inport
  wheel_rpm : Inport  Port=2
  Temp : Inport  Port=3
  Add1 : Sum
  Add2 : Sum
  Divide : Product  Inputs=/*
  Divide1 : Product  Inputs=/*
  Divide6 : Product  Inputs=*/
  Gain : Gain  Gain=2*pi/60
  Gain1 : Gain  Gain=2*pi/60
  Gearbox Ratio : Gain  Gain=config_gearbox.iges
  Lookup Gearbox : Subsystem  Variant=on
  Oilpump : Subsystem
  Product2 : Product  Inputs=**
  Saturation : Saturate  UpperLimit=inf  LowerLimit=0
  Switch2 : Switch  Criteria=u2 > Threshold  SaturateOnIntegerOverflow=off  InputSameDT=off
  Switch3 : Switch  Criteria=u2 ~= 0  SaturateOnIntegerOverflow=off  InputSameDT=off
  Switch4 : Switch  Criteria=u2 ~= 0  SaturateOnIntegerOverflow=off  InputSameDT=off
  Zero : Constant  Value=0  OutDataTypeStr=Inherit: Inherit via back propagation
  Zero1 : Constant  Value=0  OutDataTypeStr=Inherit: Inherit via back propagation
  loss_lockup : Outport
  gearbox_efficiency : Outport  Port=2
  gearbox_rpm : Outport  Port=3
  gearbox_torque : Outport  Port=4
  wires:
  Gain/1 -> Divide1/1, Divide/2, Add2/2  "wheel_power"
  wheel_torque/1 -> Lookup Gearbox/1(Torque), Product2/1  "wheel_torque"
  Lookup Gearbox/1(Loss) -> Add1/1  "powerloss_gear"
  Product2/1 -> Gain/1
  Switch4/1 -> gearbox_torque/1
  Switch3/1 -> gearbox_efficiency/1
  Gearbox Ratio/1 -> gearbox_rpm/1, Gain1/1  "gearbox_rpm"
  Switch2/1 -> Saturation/1
  Divide/1 -> Switch2/1
  Add2/1 -> Divide/1, Switch2/2, Divide1/2, Divide6/1  "gearbox_power"
  Zero/1 -> Switch4/3
  Divide6/1 -> Switch4/1
  Divide1/1 -> Switch2/3
  Oilpump/1(loss_oilpump) -> Add1/2  "powerloss_oilpump"
  Add1/1 -> loss_lockup/1, Add2/1  "powerloss_gearbox"
  Temp/1 -> Lookup Gearbox/3(Temp)
  Gain1/1 -> Switch4/2, Divide6/2
  wheel_rpm/1 -> Switch3/2, Gearbox Ratio/1, Product2/2, Lookup Gearbox/2(RPM), Oilpump/1(rpm_wheel)  "wheel_rpm"
  Zero1/1 -> Switch3/3
  Saturation/1 -> Switch3/1

== system SimulationWithMotorAndGearbox/Variant Subsystem Gearbox/Gearbox Analytic/Variant Subsystem Analytic GB/Einstufig_Achsparallel/Ölpumpe ==
  nrad : Inport
  Constant : Constant  Value=config_gearbox.power_oilpump
  Constant1 : Constant  Value=1.5e3
  Product : Product  Inputs=*/*
  Scope : Scope
  power_oilpump : Outport
  wires:
  Product/1 -> power_oilpump/1, Scope/1
  Constant1/1 -> Product/2
  nrad/1 -> Product/1
  Constant/1 -> Product/3

== system SimulationWithMotorAndGearbox/Variant Subsystem Gearbox/Gearbox Analytic/Variant Subsystem Analytic GB/Zweistufig_Achsparallel/Ölpumpe ==
  nrad : Inport
  Constant : Constant  Value=config_gearbox.power_oilpump
  Constant1 : Constant  Value=15e3
  Product : Product  Inputs=*/*
  Scope : Scope
  power_oilpump : Outport
  wires:
  Product/1 -> power_oilpump/1, Scope/1
  Constant1/1 -> Product/2
  nrad/1 -> Product/1
  Constant/1 -> Product/3

== system SimulationWithMotorAndGearbox/Variant Subsystem Gearbox/Gearbox Analytic/Variant Subsystem Analytic GB/Zweistufig_Koaxial/Ölpumpe ==
  nrad : Inport
  Constant : Constant  Value=config_gearbox.power_oilpump
  Constant1 : Constant  Value=1.5e3
  Product : Product  Inputs=*/*
  Scope : Scope
  power_oilpump : Outport
  wires:
  Product/1 -> power_oilpump/1, Scope/1
  Constant1/1 -> Product/2
  nrad/1 -> Product/1
  Constant/1 -> Product/3

== system SimulationWithMotorAndGearbox/Variant Subsystem Gearbox/Gearbox Lookup-Table/Variant Subsystem/ETA_map/Lookup Gearbox ==
  note: 1) Add Subsystem or Model blocks as valid variant choices.
      | 2) You cannot connect blocks at this level. At simulation, connectivity is automatically
      | determined, based on the active variant and port name matching.
  Torque : Inport
  RPM : Inport  Port=2
  Temp : Inport  Port=3
  Lookup with Temp : Subsystem  VariantControl=gearbox_map.dim_lookup == 3
  Lookup without Temp : Subsystem  VariantControl=gearbox_map.dim_lookup == 2
  Eta : Outport

== system SimulationWithMotorAndGearbox/Variant Subsystem Gearbox/Gearbox Lookup-Table/Variant Subsystem/ETA_map/Oilpump ==
  rpm_wheel : Inport
  Constant7 : Constant  Value=config_gearbox.power_oilpump
  Constant8 : Constant  Value=1.5e3
  Product4 : Product  Inputs=**/
  loss_oilpump : Outport
  wires:
  rpm_wheel/1 -> Product4/1
  Constant8/1 -> Product4/3
  Constant7/1 -> Product4/2
  Product4/1 -> loss_oilpump/1  "loss_oilpump"

== system SimulationWithMotorAndGearbox/Variant Subsystem Gearbox/Gearbox Lookup-Table/Variant Subsystem/LOSS_map/Lookup Gearbox ==
  note: 1) Add Subsystem or Model blocks as valid variant choices.
      | 2) You cannot connect blocks at this level. At simulation, connectivity is automatically
      | determined, based on the active variant and port name matching.
  Torque : Inport
  RPM : Inport  Port=2
  Temp : Inport  Port=3
  Lookup with Temp : Subsystem  VariantControl=gearbox_map.dim_lookup == 3
  Lookup without Temp : Subsystem  VariantControl=gearbox_map.dim_lookup == 2
  Loss : Outport

== system SimulationWithMotorAndGearbox/Variant Subsystem Gearbox/Gearbox Lookup-Table/Variant Subsystem/LOSS_map/Oilpump ==
  rpm_wheel : Inport
  Constant7 : Constant  Value=config_gearbox.power_oilpump
  Constant8 : Constant  Value=1.5e3
  Product4 : Product  Inputs=**/
  loss_oilpump : Outport
  wires:
  Product4/1 -> loss_oilpump/1  "loss_oilpump"
  Constant7/1 -> Product4/2
  Constant8/1 -> Product4/3
  rpm_wheel/1 -> Product4/1

== system SimulationWithMotorAndGearbox/Variant Subsystem Gearbox/Gearbox Lookup-Table/Variant Subsystem/ETA_map/Lookup Gearbox/Lookup with Temp ==
  Torque : Inport
  RPM : Inport  Port=2
  Temp : Inport  Port=3
  n-D Lookup Table : Lookup_n-D  NumberOfTableDimensions=3  BreakpointsForDimension1=gearbox_map.torque  BreakpointsForDimension2=gearbox_map.rpm  BreakpointsForDimension3=gearbox_map.temperature  Table=gearbox_map.eta  UseLastTableValue=on  InternalRulePriority=Speed  RndMeth=Simplest
      settings: InputPortMap=u0,u1,u2
  Eta : Outport
  wires:
  Torque/1 -> n-D Lookup Table/1
  RPM/1 -> n-D Lookup Table/2
  Temp/1 -> n-D Lookup Table/3
  n-D Lookup Table/1 -> Eta/1

== system SimulationWithMotorAndGearbox/Variant Subsystem Gearbox/Gearbox Lookup-Table/Variant Subsystem/ETA_map/Lookup Gearbox/Lookup without Temp ==
  Torque : Inport
  RPM : Inport  Port=2
  n-D Lookup Table : Lookup_n-D  BreakpointsForDimension1=gearbox_map.torque  BreakpointsForDimension2=gearbox_map.rpm  BreakpointsForDimension3=gearbox_map.temperature  Table=gearbox_map.eta  UseLastTableValue=on  InternalRulePriority=Speed  RndMeth=Simplest
      settings: InputPortMap=u0,u1
  Eta : Outport
  wires:
  Torque/1 -> n-D Lookup Table/1
  RPM/1 -> n-D Lookup Table/2
  n-D Lookup Table/1 -> Eta/1

== system SimulationWithMotorAndGearbox/Variant Subsystem Gearbox/Gearbox Lookup-Table/Variant Subsystem/LOSS_map/Lookup Gearbox/Lookup with Temp ==
  Torque : Inport
  RPM : Inport  Port=2
  Temp : Inport  Port=3
  n-D Lookup Table : Lookup_n-D  NumberOfTableDimensions=3  BreakpointsForDimension1=gearbox_map.torque  BreakpointsForDimension2=gearbox_map.rpm  BreakpointsForDimension3=gearbox_map.temperature  Table=gearbox_map.loss  UseLastTableValue=on  InternalRulePriority=Speed  RndMeth=Simplest
      settings: InputPortMap=u0,u1,u2
  Loss : Outport
  wires:
  n-D Lookup Table/1 -> Loss/1
  Temp/1 -> n-D Lookup Table/3
  RPM/1 -> n-D Lookup Table/2
  Torque/1 -> n-D Lookup Table/1

== system SimulationWithMotorAndGearbox/Variant Subsystem Gearbox/Gearbox Lookup-Table/Variant Subsystem/LOSS_map/Lookup Gearbox/Lookup without Temp ==
  Torque : Inport
  RPM : Inport  Port=2
  n-D Lookup Table : Lookup_n-D  BreakpointsForDimension1=gearbox_map.torque  BreakpointsForDimension2=gearbox_map.rpm  BreakpointsForDimension3=gearbox_map.temperature  Table=gearbox_map.loss  UseLastTableValue=on  InternalRulePriority=Speed  RndMeth=Simplest
      settings: InputPortMap=u0,u1
  Loss : Outport
  wires:
  n-D Lookup Table/1 -> Loss/1
  RPM/1 -> n-D Lookup Table/2
  Torque/1 -> n-D Lookup Table/1

== matlab function SimulationWithMotorAndGearbox/Variant Subsystem Gearbox/Gearbox Analytic/Variant Subsystem Analytic GB/Einstufig_Achsparallel/MATLAB Function ==
  data: P_V output double size=1; Mrad input; nrad input; Temp input; GB parameter
function P_V = Getriebe_Einstufig_Achsparallel(Mrad, nrad, Temp, GB)

if nrad == 0
    P_V = 0;
else
    P_V = Getrieberechnung_Einstufig(GB,Mrad,nrad);
end

end

== matlab function SimulationWithMotorAndGearbox/Variant Subsystem Gearbox/Gearbox Lookup-Table/Oil Temp/MATLAB Function ==
  data: t input; P_V input; T output
function T = fcn(t, P_V)

coder.extrinsic('evalin');

% Calculate lubricant temperature
ambient_temp = 0;
ambient_temp = evalin('base', 'config_vehicle.ambient_temp');
% 
% if t < (ambient_temp - 273)
%     T = (ambient_temp - 273);
% elseif t <= 70 %Aufwärmphase mit Umgebung < t < 70°C
%     T = abs(P) * 0.0003 + rpm * 0.00004 + t; %Leistungsabhängiger und drehzahlabhängiger Energieeintrag (Temperaturanstieg)
% else %Temperatur t > 70°C -> Wärmeabgabe ~ delta_t und ~ delta_t^2 (mit delta_t = t_gearbox - t_ambient)
%     T = abs(P) * 0.0003 + rpm * 0.00004 + t - (t - ambient_temp + 273) * 0.0002 - (t - ambient_temp + 273)^2 * 0.0000022;
% end

if t < (ambient_temp - 273)
    T = (ambient_temp - 273);
elseif t <= 80 %Aufwärmphase mit Umgebung < t < 70°C
    T =0.000055*P_V + t - (t - ambient_temp + 273) * 0.0003; %Leistungsabhängiger und drehzahlabhängiger Energieeintrag (Temperaturanstieg)
else %Temperatur t > 70°C -> Wärmeabgabe ~ delta_t und ~ delta_t^2 (mit delta_t = t_gearbox - t_ambient)
    T = 0.000088*P_V + t - (t - ambient_temp + 273) * 0.0010 - (t - ambient_temp + 273)^2 * 0.000012;
end

end

== matlab function SimulationWithMotorAndGearbox/Variant Subsystem Gearbox/Gearbox Analytic/Oil Temp/MATLAB Function ==
  data: t input; P_V input; T output
function T = fcn(t, P_V)

coder.extrinsic('evalin');

% Calculate lubricant temperature
ambient_temp = 0;
ambient_temp = evalin('base', 'config_vehicle.ambient_temp');
% 
% if t < (ambient_temp - 273)
%     T = (ambient_temp - 273);
% elseif t <= 70 %Aufwärmphase mit Umgebung < t < 70°C
%     T = abs(P) * 0.0003 + rpm * 0.00004 + t; %Leistungsabhängiger und drehzahlabhängiger Energieeintrag (Temperaturanstieg)
% else %Temperatur t > 70°C -> Wärmeabgabe ~ delta_t und ~ delta_t^2 (mit delta_t = t_gearbox - t_ambient)
%     T = abs(P) * 0.0003 + rpm * 0.00004 + t - (t - ambient_temp + 273) * 0.0002 - (t - ambient_temp + 273)^2 * 0.0000022;
% end

if t < (ambient_temp - 273)
    T = (ambient_temp - 273);
elseif t <= 80 %Aufwärmphase mit Umgebung < t < 70°C
    T =0.000055*P_V + t - (t - ambient_temp + 273) * 0.0003; %Leistungsabhängiger und drehzahlabhängiger Energieeintrag (Temperaturanstieg)
else %Temperatur t > 70°C -> Wärmeabgabe ~ delta_t und ~ delta_t^2 (mit delta_t = t_gearbox - t_ambient)
    T = 0.000088*P_V + t - (t - ambient_temp + 273) * 0.0010 - (t - ambient_temp + 273)^2 * 0.000012;
end

end

== matlab function SimulationWithMotorAndGearbox/Variant Subsystem Gearbox/Gearbox Lookup-Table/Oil Temp Gao/MATLAB Function ==
  data: t input; P input; T output; rpm input
function T = fcn(t, P, rpm)

coder.extrinsic('evalin');

% Calculate lubricant temperature
ambient_temp = 0;
ambient_temp = evalin('base', 'config_vehicle.ambient_temp');

% if t < (ambient_temp - 273)
%     T = (ambient_temp - 273);
% elseif t <= 75
%     T = abs(P) * 0.005 + t - (t - ambient_temp + 273)* 0.001;
% else
%     T = abs(P) * 0.005 + t - (t - 75) * 0.002 - (t - ambient_temp + 273)* 0.001;
% end

if t < (ambient_temp - 273)
    T = (ambient_temp - 273);
elseif t <= 70 %Aufwärmphase mit Umgebung < t < 70°C
    T = abs(P) * 0.0003 + rpm * 0.00004 + t; %Leistungsabhängiger und drehzahlabhängiger Energieeintrag (Temperaturanstieg)
else %Temperatur t > 70°C -> Wärmeabgabe ~ delta_t und ~ delta_t^2 (mit delta_t = t_gearbox - t_ambient)
    T = abs(P) * 0.0003 + rpm * 0.00004 + t - (t - ambient_temp + 273) * 0.0002 - (t - ambient_temp + 273)^2 * 0.0000022;
end

end

== matlab function SimulationWithMotorAndGearbox/Variant Subsystem Gearbox/Gearbox Analytic/Variant Subsystem Analytic GB/Zweistufig_Koaxial/MATLAB Function ==
  data: P_V output double size=1; Mrad input; nrad input; Temp input; GB parameter
function P_V = Getriebe_Einstufig_Achsparallel(Mrad, nrad, Temp, GB)

if nrad == 0
    P_V = 0;
else
    P_V = Getrieberechnung_koaxial(GB,Mrad,nrad,Temp);
end

end

== matlab function SimulationWithMotorAndGearbox/Variant Subsystem Gearbox/Gearbox Analytic/Oil Temp Gao/MATLAB Function ==
  data: t input; P input; T output; rpm input
function T = fcn(t, P, rpm)

coder.extrinsic('evalin');

% Calculate lubricant temperature
ambient_temp = 0;
ambient_temp = evalin('base', 'config_vehicle.ambient_temp');

% if t < (ambient_temp - 273)
%     T = (ambient_temp - 273);
% elseif t <= 75
%     T = abs(P) * 0.005 + t - (t - ambient_temp + 273)* 0.001;
% else
%     T = abs(P) * 0.005 + t - (t - 75) * 0.002 - (t - ambient_temp + 273)* 0.001;
% end

if t < (ambient_temp - 273)
    T = (ambient_temp - 273);
elseif t <= 70 %Aufwärmphase mit Umgebung < t < 70°C
    T = abs(P) * 0.0003 + rpm * 0.00004 + t; %Leistungsabhängiger und drehzahlabhängiger Energieeintrag (Temperaturanstieg)
else %Temperatur t > 70°C -> Wärmeabgabe ~ delta_t und ~ delta_t^2 (mit delta_t = t_gearbox - t_ambient)
    T = abs(P) * 0.0003 + rpm * 0.00004 + t - (t - ambient_temp + 273) * 0.0002 - (t - ambient_temp + 273)^2 * 0.0000022;
end

end

== matlab function SimulationWithMotorAndGearbox/Variant Subsystem Gearbox/Gearbox Analytic/Variant Subsystem Analytic GB/Zweistufig_Achsparallel/MATLAB Function ==
  data: P_V output double size=1; Mrad input; nrad input; Temp input; GB parameter
function P_V  = Getriebe_Zweistufig_Achsparallel(Mrad, nrad, Temp, GB)

if nrad == 0
    P_V = 0;
else
    [P_V] = Getrieberechnung(GB,Mrad,nrad,Temp);
end

end

== matlab function SimulationWithMotorAndGearbox/Variant Subsystem Motor/Motor Lookup-TableOneMotor/MATLAB Function2 ==
  data: u input; y output
function y = fcn(u)

if isnan(u)
    %warning('P_motor_111 is NaN. Setting it to 0.');
    y = 0;
else
    y = u;
end
